simulink model "mrefrobotarm_modified_previous_y_previous_u_previous_ref"  (R2018b)
settings: Solver=FixedStepAuto  StartTime=0.0  StopTime=10  RelTol=1e-3  AbsTol=1e-6
undefined symbols (not defined in the file or in its folder): options, sfunxy2
libraries: neural x949, simulink x1
(part 8 of 31)

== system mrefrobotarm_modified_previous_y_previous_u_previous_ref/Feed-Forward Neural Network/Layer 2/Delays 1 ==
  "p{2}" : Inport  PortDimensions=60
      mask Display: e = 0.06;c1 = [120 230 180]/255;c2 = ([120 230 180]+0)/(256+128);c3 = ([120 230 180]+128)/(256+128);patch([0 1 1 0],[0 0 1 1],c1);patch([0 1 1 1-e 1-e 0+e],[0 0 1 1-e 0+e 0+e],c2);patch([0 0 1 1-e 0+e 0+e],[0 1 1 1-e 1-e 0+e],c3);plot([0 1 1 0 0],[0 0 1 1 0]);
  mux : Mux  Inputs=1
      mask Display: e = 0.06;c1 = [120 150 230]/255;c2 = ([120 150 230]+0)/383;c3 = ([120 150 230]+128)/383;patch([0 1 1 0],[0 0 1 1],c1);patch([0 1 1 1-e 1-e 0+e],[0 0 1 1-e 0+e 0+e],c2);patch([0 0 1 1-e 0+e 0+e],[0 1 1 1-e 1-e 0+e],c3);plot([0 1 1 0 0],[0 0 1 1 0]);disp('Mux')
  "pd{2,1}" : Outport
      mask Display: e = 0.06;c1 = [120 230 180]/255;c2 = ([120 230 180]+0)/(256+128);c3 = ([120 230 180]+128)/(256+128);patch([0 1 1 0],[0 0 1 1],c1);patch([0 1 1 1-e 1-e 0+e],[0 0 1 1-e 0+e 0+e],c2);patch([0 0 1 1-e 0+e 0+e],[0 1 1 1-e 1-e 0+e],c3);plot([0 1 1 0 0],[0 0 1 1 0]);
  wires:
  "p{2}"/1 -> mux/1
  mux/1 -> "pd{2,1}"/1

== system mrefrobotarm_modified_previous_y_previous_u_previous_ref/Feed-Forward Neural Network/Layer 2/LW{2,1} ==
  "ad{2,1}" : Inport  PortDimensions=60
      mask Display: e = 0.06;c1 = [120 230 180]/255;c2 = ([120 230 180]+0)/(256+128);c3 = ([120 230 180]+128)/(256+128);patch([0 1 1 0],[0 0 1 1],c1);patch([0 1 1 1-e 1-e 0+e],[0 0 1 1-e 0+e 0+e],c2);patch([0 0 1 1-e 0+e 0+e],[0 1 1 1-e 1-e 0+e],c3);plot([0 1 1 0 0],[0 0 1 1 0]);
  "IW{2,1}(1,:)'" : Constant  Value=[0.004922335615622427072712863349579492933116853237152099609375;-0.000568123825967846766103741540376859120442532002925872802734375;-0.088069540363433007623683579367934726178646087646484375;0.008040519008257716870868847536257817409932613372802734375;-1.1046255112634393302784019397222436964511871337890625;1.0155388829671150308087135272216983139514923095703125;-0.0584137446587948971910009277053177356719970703125;-0.60279808328518191817835258916602469980716705322265625;-0.002127023321206248686332518360586618655361235141754150390625;-0.702093460779070976940374748664908111095428466796875;-0.5646190112434352759152034195722080767154693603515625;0.1977466023732981081906245890422724187374114990234375;0.053988746168900279831515121031770831905305385589599609375;-0.0836139079239973381785233641494414769113063812255859375;0.000321793533986787310373356429948898949078284204006195068359375;0.01929470514180042783891622093506157398223876953125;-0.004037426007550685112812427490780464722774922847747802734375;-0.006774271389454964049925411728736435179598629474639892578125;-0.12049917647571557755004079126592841930687427520751953125;-0.274181794734965844639873466803692281246185302734375;-0.03381345636772016549631558746114023961126804351806640625;-0.084568291882440027595890796874300576746463775634765625;0.01009376083310289419492367102293428615666925907135009765625;-0.1481308970879313402502219787493231706321239471435546875;-1.83977190390720490853482260718010365962982177734375;-0.0309407696275533876384411513527084025554358959197998046875;0.2451901685169690370269535151237505488097667694091796875;0.11553958397011880598892474836247856728732585906982421875;0.004316504239658881802998990906417020596563816070556640625;0.38419726481958960118134882577578537166118621826171875;-0.036990773747104264967955344900474301539361476898193359375;0.05294928752338227961882211047850432805716991424560546875;-0.004316566647762872833971048436296769068576395511627197265625;-0.00471011047120292215828474269301295862533152103424072265625;0.86826225761141750947302853091969154775142669677734375;-0.272835736891962998829086473051575012505054473876953125;-0.0133865280367646798109770855944589129649102687835693359375;0.56412398957959453138499839042196981608867645263671875;-0.4238701061208143272551751579158008098602294921875;-0.0239428666309109867971205432013448444195091724395751953125;-1.46284474525641439157652712310664355754852294921875;-0.01846824999686343116156450605558347888290882110595703125;-1.8796503475121746351561569099430926144123077392578125;0.5565875164302613864464319703984074294567108154296875;-1.2035129714628267638687475482583977282047271728515625;-0.396624881636485737690378527986467815935611724853515625;0.374562923409318404566192839411087334156036376953125;0.228885480374885597054657182525261305272579193115234375;0.29055525212637800525072862001252360641956329345703125;-0.01447757195351602292621162604291384923271834850311279296875;-0.0176065930859190811208492277728510089218616485595703125;-0.2212805191454988718025020943969138897955417633056640625;-0.064717987937388699037910555489361286163330078125;-0.402780257895579529847651656382367946207523345947265625;0.89397582203941539091829326935112476348876953125;-0.156302033504358173221504557659500278532505035400390625;-0.0055868107216290908978439944121419102884829044342041015625;-0.34665630432465055488222560597932897508144378662109375;-0.206360303612080742130530097711016424000263214111328125;0.35959441595475760689026856198324821889400482177734375]
      mask Display: e = 0.06;c1 = [120 150 230]/255;c2 = ([120 150 230]+0)/383;c3 = ([120 150 230]+128)/383;patch([0 1 1 0],[0 0 1 1],c1);patch([0 1 1 1-e 1-e 0+e],[0 0 1 1-e 0+e 0+e],c2);patch([0 0 1 1-e 0+e 0+e],[0 1 1 1-e 1-e 0+e],c3);plot([0 1 1 0 0],[0 0 1 1 0]);disp('weights');
  Mux : Mux  Inputs=1
      mask Display: e = 0.06;c1 = [120 150 230]/255;c2 = ([120 150 230]+0)/383;c3 = ([120 150 230]+128)/383;patch([0 1 1 0],[0 0 1 1],c1);patch([0 1 1 1-e 1-e 0+e],[0 0 1 1-e 0+e 0+e],c2);patch([0 0 1 1-e 0+e 0+e],[0 1 1 1-e 1-e 0+e],c3);plot([0 1 1 0 0],[0 0 1 1 0]);disp('Mux');
  dotprod1 : neural/Weight Functions/dotprod
  "lz{2,1}" : Outport
      mask Display: e = 0.06;c1 = [120 230 180]/255;c2 = ([120 230 180]+0)/(256+128);c3 = ([120 230 180]+128)/(256+128);patch([0 1 1 0],[0 0 1 1],c1);patch([0 1 1 1-e 1-e 0+e],[0 0 1 1-e 0+e 0+e],c2);patch([0 0 1 1-e 0+e 0+e],[0 1 1 1-e 1-e 0+e],c3);plot([0 1 1 0 0],[0 0 1 1 0]);
  wires:
  "IW{2,1}(1,:)'"/1 -> dotprod1/1
  "ad{2,1}"/1 -> dotprod1/2
  dotprod1/1 -> Mux/1
  Mux/1 -> "lz{2,1}"/1

== system mrefrobotarm_modified_previous_y_previous_u_previous_ref/Feed-Forward Neural Network1/Layer 1/Delays 1 ==
  "p{1}" : Inport  PortDimensions=8
      mask Display: e = 0.06;c1 = [120 230 180]/255;c2 = ([120 230 180]+0)/(256+128);c3 = ([120 230 180]+128)/(256+128);patch([0 1 1 0],[0 0 1 1],c1);patch([0 1 1 1-e 1-e 0+e],[0 0 1 1-e 0+e 0+e],c2);patch([0 0 1 1-e 0+e 0+e],[0 1 1 1-e 1-e 0+e],c3);plot([0 1 1 0 0],[0 0 1 1 0]);
  mux : Mux  Inputs=1
      mask Display: e = 0.06;c1 = [120 150 230]/255;c2 = ([120 150 230]+0)/383;c3 = ([120 150 230]+128)/383;patch([0 1 1 0],[0 0 1 1],c1);patch([0 1 1 1-e 1-e 0+e],[0 0 1 1-e 0+e 0+e],c2);patch([0 0 1 1-e 0+e 0+e],[0 1 1 1-e 1-e 0+e],c3);plot([0 1 1 0 0],[0 0 1 1 0]);disp('Mux')
  "pd{1,1}" : Outport
      mask Display: e = 0.06;c1 = [120 230 180]/255;c2 = ([120 230 180]+0)/(256+128);c3 = ([120 230 180]+128)/(256+128);patch([0 1 1 0],[0 0 1 1],c1);patch([0 1 1 1-e 1-e 0+e],[0 0 1 1-e 0+e 0+e],c2);patch([0 0 1 1-e 0+e 0+e],[0 1 1 1-e 1-e 0+e],c3);plot([0 1 1 0 0],[0 0 1 1 0]);
  wires:
  "p{1}"/1 -> mux/1
  mux/1 -> "pd{1,1}"/1

== system mrefrobotarm_modified_previous_y_previous_u_previous_ref/Feed-Forward Neural Network1/Layer 1/IW{1,1} ==
  "pd{1,1}" : Inport  PortDimensions=8
      mask Display: e = 0.06;c1 = [120 230 180]/255;c2 = ([120 230 180]+0)/(256+128);c3 = ([120 230 180]+128)/(256+128);patch([0 1 1 0],[0 0 1 1],c1);patch([0 1 1 1-e 1-e 0+e],[0 0 1 1-e 0+e 0+e],c2);patch([0 0 1 1-e 0+e 0+e],[0 1 1 1-e 1-e 0+e],c3);plot([0 1 1 0 0],[0 0 1 1 0]);
  "IW{1,1}(1,:)'" : Constant  Value=[-0.489435165671598337855385807415586896240711212158203125;-0.59790642458332443620605545220314525067806243896484375;0.9462514542685998009119430207647383213043212890625;0.87465564536648532367735242587514221668243408203125;-1.4123419584819483230120340522262267768383026123046875;0.364318026214990597910770020462223328649997711181640625;0.476243895384673543436093723357771523296833038330078125;-0.94161424505193591638629868612042628228664398193359375]
      mask Display: e = 0.06;c1 = [120 150 230]/255;c2 = ([120 150 230]+0)/383;c3 = ([120 150 230]+128)/383;patch([0 1 1 0],[0 0 1 1],c1);patch([0 1 1 1-e 1-e 0+e],[0 0 1 1-e 0+e 0+e],c2);patch([0 0 1 1-e 0+e 0+e],[0 1 1 1-e 1-e 0+e],c3);plot([0 1 1 0 0],[0 0 1 1 0]);disp('Weights');
  "IW{1,1}(10,:)'" : Constant  Value=[0.24784818454698787082435273987357504665851593017578125;0.428137490507039142340062198854866437613964080810546875;-0.279368989082627694475746693569817580282688140869140625;0.635561926772618246417323462083004415035247802734375;-0.2661724130434099944153558681136928498744964599609375;0.84937640623256982497224498729337938129901885986328125;1.1481977763386710389426070832996629178524017333984375;0.1470300152897714152100405726741882972419261932373046875]
      mask Display: e = 0.06;c1 = [120 150 230]/255;c2 = ([120 150 230]+0)/383;c3 = ([120 150 230]+128)/383;patch([0 1 1 0],[0 0 1 1],c1);patch([0 1 1 1-e 1-e 0+e],[0 0 1 1-e 0+e 0+e],c2);patch([0 0 1 1-e 0+e 0+e],[0 1 1 1-e 1-e 0+e],c3);plot([0 1 1 0 0],[0 0 1 1 0]);disp('Weights');
  "IW{1,1}(11,:)'" : Constant  Value=[0.4509913927567001934448853717185556888580322265625;0.7052495398937128623373382652061991393566131591796875;-0.7838302343464118582261335177463479340076446533203125;1.4900741834051085543677572786691598594188690185546875;-0.527849453687423864067795875598676502704620361328125;-1.02175108583142648654984441236592829227447509765625;-0.52620304449603716445693635250790975987911224365234375;-0.6238002211724491541389170379261486232280731201171875]
      mask Display: e = 0.06;c1 = [120 150 230]/255;c2 = ([120 150 230]+0)/383;c3 = ([120 150 230]+128)/383;patch([0 1 1 0],[0 0 1 1],c1);patch([0 1 1 1-e 1-e 0+e],[0 0 1 1-e 0+e 0+e],c2);patch([0 0 1 1-e 0+e 0+e],[0 1 1 1-e 1-e 0+e],c3);plot([0 1 1 0 0],[0 0 1 1 0]);disp('Weights');
  "IW{1,1}(12,:)'" : Constant  Value=[-1.6021052877080024234857091869344003498554229736328125;-0.400230307522328410119172303893719799816608428955078125;0.77757489461041362499571505395579151809215545654296875;0.2472458939471125216602587215675157494843006134033203125;-0.1976112083793134244213973715886822901666164398193359375;0.04669389623471220662764835651614703238010406494140625;0.511283230600608984417476676753722131252288818359375;-0.469639748921519550872716308731469325721263885498046875]
      mask Display: e = 0.06;c1 = [120 150 230]/255;c2 = ([120 150 230]+0)/383;c3 = ([120 150 230]+128)/383;patch([0 1 1 0],[0 0 1 1],c1);patch([0 1 1 1-e 1-e 0+e],[0 0 1 1-e 0+e 0+e],c2);patch([0 0 1 1-e 0+e 0+e],[0 1 1 1-e 1-e 0+e],c3);plot([0 1 1 0 0],[0 0 1 1 0]);disp('Weights');
  "IW{1,1}(13,:)'" : Constant  Value=[-1.6051933424153304041936962676118128001689910888671875;-1.5266914996233234003142342771752737462520599365234375;0.332608030744975857739831326398416422307491302490234375;-0.59175031390800969521848173826583661139011383056640625;0.45672389039967864476921022287569940090179443359375;-0.1611477461390518894912560199372819624841213226318359375;0.0258266856071377344516992735634630662389099597930908203125;1.0826091475290675614218116606934927403926849365234375]
      mask Display: e = 0.06;c1 = [120 150 230]/255;c2 = ([120 150 230]+0)/383;c3 = ([120 150 230]+128)/383;patch([0 1 1 0],[0 0 1 1],c1);patch([0 1 1 1-e 1-e 0+e],[0 0 1 1-e 0+e 0+e],c2);patch([0 0 1 1-e 0+e 0+e],[0 1 1 1-e 1-e 0+e],c3);plot([0 1 1 0 0],[0 0 1 1 0]);disp('Weights');
  "IW{1,1}(14,:)'" : Constant  Value=[-0.20824009402255339029608194323373027145862579345703125;-0.63002483804711406634169179596938192844390869140625;0.6012849457953872711613030332955531775951385498046875;0.1919364347106604640202931477688252925872802734375;-0.56970968188246418062448128694086335599422454833984375;0.2051097651594903925609258976692217402160167694091796875;0.260356801348437638665700433193705976009368896484375;1.5726063671236916174933639922528527677059173583984375]
      mask Display: e = 0.06;c1 = [120 150 230]/255;c2 = ([120 150 230]+0)/383;c3 = ([120 150 230]+128)/383;patch([0 1 1 0],[0 0 1 1],c1);patch([0 1 1 1-e 1-e 0+e],[0 0 1 1-e 0+e 0+e],c2);patch([0 0 1 1-e 0+e 0+e],[0 1 1 1-e 1-e 0+e],c3);plot([0 1 1 0 0],[0 0 1 1 0]);disp('Weights');
  "IW{1,1}(15,:)'" : Constant  Value=[0.6453341252687445628311024847789667546749114990234375;-0.5310115058985160896298793886671774089336395263671875;-0.48721002209239483438096840473008342087268829345703125;-0.63616173475083803712237795480177737772464752197265625;-0.455222345196995281657592613555607385933399200439453125;-0.20214300406766472217867658400791697204113006591796875;0.85975492967386080156444450039998628199100494384765625;-0.30000078268944407877683033802895806729793548583984375]
      mask Display: e = 0.06;c1 = [120 150 230]/255;c2 = ([120 150 230]+0)/383;c3 = ([120 150 230]+128)/383;patch([0 1 1 0],[0 0 1 1],c1);patch([0 1 1 1-e 1-e 0+e],[0 0 1 1-e 0+e 0+e],c2);patch([0 0 1 1-e 0+e 0+e],[0 1 1 1-e 1-e 0+e],c3);plot([0 1 1 0 0],[0 0 1 1 0]);disp('Weights');
  "IW{1,1}(16,:)'" : Constant  Value=[-1.2705032748254423413669655928970314562320709228515625;0.460182504971557937434312179902917705476284027099609375;-0.7014528933886319261858943718834780156612396240234375;-1.3600973186092204514352488331496715545654296875;-0.380943287230387894748417920709471218287944793701171875;-0.182287628267785828395375347099616192281246185302734375;0.76493247291822685784978830270119942724704742431640625;-0.1468958452647432244564384973273263312876224517822265625]
      mask Display: e = 0.06;c1 = [120 150 230]/255;c2 = ([120 150 230]+0)/383;c3 = ([120 150 230]+128)/383;patch([0 1 1 0],[0 0 1 1],c1);patch([0 1 1 1-e 1-e 0+e],[0 0 1 1-e 0+e 0+e],c2);patch([0 0 1 1-e 0+e 0+e],[0 1 1 1-e 1-e 0+e],c3);plot([0 1 1 0 0],[0 0 1 1 0]);disp('Weights');
  "IW{1,1}(2,:)'" : Constant  Value=[0.05544360121873585789398219958457048051059246063232421875;-0.6084945450961765089914479176513850688934326171875;0.8236590711365157080336985018220730125904083251953125;0.0942136023378637166292293159131077118217945098876953125;-0.10857743809028670700644880753316101618111133575439453125;0.02981406738831320069049723997522960416972637176513671875;0.198421637732602185177910314450855366885662078857421875;1.001382968907298387506443759775720536708831787109375]
      mask Display: e = 0.06;c1 = [120 150 230]/255;c2 = ([120 150 230]+0)/383;c3 = ([120 150 230]+128)/383;patch([0 1 1 0],[0 0 1 1],c1);patch([0 1 1 1-e 1-e 0+e],[0 0 1 1-e 0+e 0+e],c2);patch([0 0 1 1-e 0+e 0+e],[0 1 1 1-e 1-e 0+e],c3);plot([0 1 1 0 0],[0 0 1 1 0]);disp('Weights');
  "IW{1,1}(3,:)'" : Constant  Value=[-0.293870924391490262461701377105782739818096160888671875;0.48987560205334046425917904343805275857448577880859375;-0.226064051583725611482833528498304076492786407470703125;0.54526247608860656246321241269470192492008209228515625;-1.0762508709854230470881475412170402705669403076171875;0.54304733376469815908649252378381788730621337890625;0.0237025381828885155222064184954433585517108440399169921875;-0.476213427298837921330942890563164837658405303955078125]
      mask Display: e = 0.06;c1 = [120 150 230]/255;c2 = ([120 150 230]+0)/383;c3 = ([120 150 230]+128)/383;patch([0 1 1 0],[0 0 1 1],c1);patch([0 1 1 1-e 1-e 0+e],[0 0 1 1-e 0+e 0+e],c2);patch([0 0 1 1-e 0+e 0+e],[0 1 1 1-e 1-e 0+e],c3);plot([0 1 1 0 0],[0 0 1 1 0]);disp('Weights');
  "IW{1,1}(4,:)'" : Constant  Value=[1.46243602440109743412222087499685585498809814453125;-0.6143515017476561812515001292922534048557281494140625;-0.813339714393659818369997083209455013275146484375;0.12431520627244212195972039580738055519759654998779296875;1.0257454781333077420413246727548539638519287109375;-1.3024201622922590981801249654381535947322845458984375;0.57650698104107267472073772296425886452198028564453125;0.20537346279362023171444207036984153091907501220703125]
      mask Display: e = 0.06;c1 = [120 150 230]/255;c2 = ([120 150 230]+0)/383;c3 = ([120 150 230]+128)/383;patch([0 1 1 0],[0 0 1 1],c1);patch([0 1 1 1-e 1-e 0+e],[0 0 1 1-e 0+e 0+e],c2);patch([0 0 1 1-e 0+e 0+e],[0 1 1 1-e 1-e 0+e],c3);plot([0 1 1 0 0],[0 0 1 1 0]);disp('Weights');
  "IW{1,1}(5,:)'" : Constant  Value=[0.2161689026789992140731300196421216242015361785888671875;-1.068678632626362201563097187317907810211181640625;0.57330147110937723642365426712785847485065460205078125;0.08697750843062114489701031061485991813242435455322265625;-0.325667357124172607285572667024098336696624755859375;-0.04243784278384317432131211944579263217747211456298828125;1.123940770278660128411729601793922483921051025390625;1.3019794387795020629283726520952768623828887939453125]
      mask Display: e = 0.06;c1 = [120 150 230]/255;c2 = ([120 150 230]+0)/383;c3 = ([120 150 230]+128)/383;patch([0 1 1 0],[0 0 1 1],c1);patch([0 1 1 1-e 1-e 0+e],[0 0 1 1-e 0+e 0+e],c2);patch([0 0 1 1-e 0+e 0+e],[0 1 1 1-e 1-e 0+e],c3);plot([0 1 1 0 0],[0 0 1 1 0]);disp('Weights');
  "IW{1,1}(6,:)'" : Constant  Value=[-1.2478069984792659052885710480040870606899261474609375;-0.1258253740427072997487556449414114467799663543701171875;-0.88679456135978573794176327282912097871303558349609375;-0.2182788795135275072833991316656465642154216766357421875;-0.7833970842850959126479892802308313548564910888671875;0.9419426170986813229291101379203610122203826904296875;-1.05803585202793914987751122680492699146270751953125;0.9246942036142489218519813221064396202564239501953125]
      mask Display: e = 0.06;c1 = [120 150 230]/255;c2 = ([120 150 230]+0)/383;c3 = ([120 150 230]+128)/383;patch([0 1 1 0],[0 0 1 1],c1);patch([0 1 1 1-e 1-e 0+e],[0 0 1 1-e 0+e 0+e],c2);patch([0 0 1 1-e 0+e 0+e],[0 1 1 1-e 1-e 0+e],c3);plot([0 1 1 0 0],[0 0 1 1 0]);disp('Weights');
  "IW{1,1}(7,:)'" : Constant  Value=[1.59052415695107551840692394762299954891204833984375;-1.407606543352498018606411278597079217433929443359375;-0.33944053433563514676762906674412079155445098876953125;-0.72464187144598124490357804461382329463958740234375;1.7120549882542188679934724859776906669139862060546875;-0.74145695282181967034063063692883588373661041259765625;0.50968036339168032444746359033160842955112457275390625;0.83650127749657865461330175094190053641796112060546875]
      mask Display: e = 0.06;c1 = [120 150 230]/255;c2 = ([120 150 230]+0)/383;c3 = ([120 150 230]+128)/383;patch([0 1 1 0],[0 0 1 1],c1);patch([0 1 1 1-e 1-e 0+e],[0 0 1 1-e 0+e 0+e],c2);patch([0 0 1 1-e 0+e 0+e],[0 1 1 1-e 1-e 0+e],c3);plot([0 1 1 0 0],[0 0 1 1 0]);disp('Weights');
  "IW{1,1}(8,:)'" : Constant  Value=[0.0659504331933596088521909450719249434769153594970703125;-0.98697499307263447665405919906334020197391510009765625;1.1401596825984083860561213441542349755764007568359375;-1.0640028818961406731347096865647472441196441650390625;-0.4904056650842238962439978422480635344982147216796875;-0.361254192958798736601266909929108805954456329345703125;-0.41512670811280916183250155881978571414947509765625;-0.43991779302995437372914011575630865991115570068359375]
      mask Display: e = 0.06;c1 = [120 150 230]/255;c2 = ([120 150 230]+0)/383;c3 = ([120 150 230]+128)/383;patch([0 1 1 0],[0 0 1 1],c1);patch([0 1 1 1-e 1-e 0+e],[0 0 1 1-e 0+e 0+e],c2);patch([0 0 1 1-e 0+e 0+e],[0 1 1 1-e 1-e 0+e],c3);plot([0 1 1 0 0],[0 0 1 1 0]);disp('Weights');
  "IW{1,1}(9,:)'" : Constant  Value=[0.9288936158440825874293977904017083346843719482421875;0.1536580527370895177252663188482983969151973724365234375;-1.1504658879815246041999898807262070477008819580078125;-0.5619971281848823441151807855931110680103302001953125;-0.304875849992781444708356275441474281251430511474609375;-0.857832390191720417504939177888445556163787841796875;0.6730201883496238490778296181815676391124725341796875;0.330856347068350709061945735811605118215084075927734375]
      mask Display: e = 0.06;c1 = [120 150 230]/255;c2 = ([120 150 230]+0)/383;c3 = ([120 150 230]+128)/383;patch([0 1 1 0],[0 0 1 1],c1);patch([0 1 1 1-e 1-e 0+e],[0 0 1 1-e 0+e 0+e],c2);patch([0 0 1 1-e 0+e 0+e],[0 1 1 1-e 1-e 0+e],c3);plot([0 1 1 0 0],[0 0 1 1 0]);disp('Weights');
  Mux : Mux  Inputs=16
      mask Display: e = 0.06;c1 = [120 150 230]/255;c2 = ([120 150 230]+0)/383;c3 = ([120 150 230]+128)/383;patch([0 1 1 0],[0 0 1 1],c1);patch([0 1 1 1-e 1-e 0+e],[0 0 1 1-e 0+e 0+e],c2);patch([0 0 1 1-e 0+e 0+e],[0 1 1 1-e 1-e 0+e],c3);plot([0 1 1 0 0],[0 0 1 1 0]);disp('Mux');
  dotprod{1..16} (16 alike) : neural/Weight Functions/dotprod
  "iz{1,1}" : Outport
      mask Display: e = 0.06;c1 = [120 230 180]/255;c2 = ([120 230 180]+0)/(256+128);c3 = ([120 230 180]+128)/(256+128);patch([0 1 1 0],[0 0 1 1],c1);patch([0 1 1 1-e 1-e 0+e],[0 0 1 1-e 0+e 0+e],c2);patch([0 0 1 1-e 0+e 0+e],[0 1 1 1-e 1-e 0+e],c3);plot([0 1 1 0 0],[0 0 1 1 0]);
  wires:
  "IW{1,1}(1,:)'"/1 -> dotprod1/1
  "pd{1,1}"/1 -> dotprod1/2, dotprod2/2, dotprod3/2, dotprod4/2, dotprod5/2, dotprod6/2, dotprod7/2, dotprod8/2, dotprod9/2, dotprod10/2, dotprod11/2, dotprod12/2, dotprod13/2, dotprod14/2, dotprod15/2, dotprod16/2
  dotprod1/1 -> Mux/1
  "IW{1,1}(2,:)'"/1 -> dotprod2/1
  dotprod2/1 -> Mux/2
  "IW{1,1}(3,:)'"/1 -> dotprod3/1
  dotprod3/1 -> Mux/3
  "IW{1,1}(4,:)'"/1 -> dotprod4/1
  dotprod4/1 -> Mux/4
  "IW{1,1}(5,:)'"/1 -> dotprod5/1
  dotprod5/1 -> Mux/5
  "IW{1,1}(6,:)'"/1 -> dotprod6/1
  dotprod6/1 -> Mux/6
  "IW{1,1}(7,:)'"/1 -> dotprod7/1
  dotprod7/1 -> Mux/7
  "IW{1,1}(8,:)'"/1 -> dotprod8/1
  dotprod8/1 -> Mux/8
  "IW{1,1}(9,:)'"/1 -> dotprod9/1
  dotprod9/1 -> Mux/9
  "IW{1,1}(10,:)'"/1 -> dotprod10/1
  dotprod10/1 -> Mux/10
  "IW{1,1}(11,:)'"/1 -> dotprod11/1
  dotprod11/1 -> Mux/11
  "IW{1,1}(12,:)'"/1 -> dotprod12/1
  dotprod12/1 -> Mux/12
  "IW{1,1}(13,:)'"/1 -> dotprod13/1
  dotprod13/1 -> Mux/13
  "IW{1,1}(14,:)'"/1 -> dotprod14/1
  dotprod14/1 -> Mux/14
  "IW{1,1}(15,:)'"/1 -> dotprod15/1
  dotprod15/1 -> Mux/15
  "IW{1,1}(16,:)'"/1 -> dotprod16/1
  dotprod16/1 -> Mux/16
  Mux/1 -> "iz{1,1}"/1

== system mrefrobotarm_modified_previous_y_previous_u_previous_ref/Feed-Forward Neural Network1/Layer 2/Delays 1 ==
  "p{2}" : Inport  PortDimensions=16
      mask Display: e = 0.06;c1 = [120 230 180]/255;c2 = ([120 230 180]+0)/(256+128);c3 = ([120 230 180]+128)/(256+128);patch([0 1 1 0],[0 0 1 1],c1);patch([0 1 1 1-e 1-e 0+e],[0 0 1 1-e 0+e 0+e],c2);patch([0 0 1 1-e 0+e 0+e],[0 1 1 1-e 1-e 0+e],c3);plot([0 1 1 0 0],[0 0 1 1 0]);
  mux : Mux  Inputs=1
      mask Display: e = 0.06;c1 = [120 150 230]/255;c2 = ([120 150 230]+0)/383;c3 = ([120 150 230]+128)/383;patch([0 1 1 0],[0 0 1 1],c1);patch([0 1 1 1-e 1-e 0+e],[0 0 1 1-e 0+e 0+e],c2);patch([0 0 1 1-e 0+e 0+e],[0 1 1 1-e 1-e 0+e],c3);plot([0 1 1 0 0],[0 0 1 1 0]);disp('Mux')
  "pd{2,1}" : Outport
      mask Display: e = 0.06;c1 = [120 230 180]/255;c2 = ([120 230 180]+0)/(256+128);c3 = ([120 230 180]+128)/(256+128);patch([0 1 1 0],[0 0 1 1],c1);patch([0 1 1 1-e 1-e 0+e],[0 0 1 1-e 0+e 0+e],c2);patch([0 0 1 1-e 0+e 0+e],[0 1 1 1-e 1-e 0+e],c3);plot([0 1 1 0 0],[0 0 1 1 0]);
  wires:
  "p{2}"/1 -> mux/1
  mux/1 -> "pd{2,1}"/1

== system mrefrobotarm_modified_previous_y_previous_u_previous_ref/Feed-Forward Neural Network1/Layer 2/LW{2,1} ==
  "ad{2,1}" : Inport  PortDimensions=16
      mask Display: e = 0.06;c1 = [120 230 180]/255;c2 = ([120 230 180]+0)/(256+128);c3 = ([120 230 180]+128)/(256+128);patch([0 1 1 0],[0 0 1 1],c1);patch([0 1 1 1-e 1-e 0+e],[0 0 1 1-e 0+e 0+e],c2);patch([0 0 1 1-e 0+e 0+e],[0 1 1 1-e 1-e 0+e],c3);plot([0 1 1 0 0],[0 0 1 1 0]);
  "IW{2,1}(1,:)'" : Constant  Value=[-0.11795628438408246874136153792278491891920566558837890625;-0.7266789733215304192270878047565929591655731201171875;-0.01225474918483036683436449010287105920724570751190185546875;1.02269129686591053740585266496054828166961669921875;0.5591836780849244181723634028458036482334136962890625;0.42706217586793082663376708296709693968296051025390625;-0.417388293832526124926829425021423958241939544677734375;-0.1721134449178444991712666478633764199912548065185546875;0.6953623528184278423935893442831002175807952880859375;0.5549726126551786098417551329475827515125274658203125;-0.75980368835832035045996235567145049571990966796875;-0.12272926696519197153900648800117778591811656951904296875;-0.42041936020313819266647215044940821826457977294921875;0.20980740921632012874198380814050324261188507080078125;-0.5296127441355171772130461249616928398609161376953125;0.2295249142940899156339895625933422707021236419677734375]
      mask Display: e = 0.06;c1 = [120 150 230]/255;c2 = ([120 150 230]+0)/383;c3 = ([120 150 230]+128)/383;patch([0 1 1 0],[0 0 1 1],c1);patch([0 1 1 1-e 1-e 0+e],[0 0 1 1-e 0+e 0+e],c2);patch([0 0 1 1-e 0+e 0+e],[0 1 1 1-e 1-e 0+e],c3);plot([0 1 1 0 0],[0 0 1 1 0]);disp('weights');
  "IW{2,1}(2,:)'" : Constant  Value=[-0.70693226414642784671826802878058515489101409912109375;0.256775847609288121464743426258792169392108917236328125;-0.94969196839098402040946211855043657124042510986328125;-0.424726446476546837249799182245624251663684844970703125;0.11347593592205339196876678897751844488084316253662109375;0.008291581221170109261553449186976649798452854156494140625;0.1784639836572024240712863729640957899391651153564453125;0.01066492483621101113044904451498950948007404804229736328125;-0.00995209252704191103811037777404635562561452388763427734375;-0.00229363338981328386545488484671295736916363239288330078125;-0.0224035193360632121917230819008182152174413204193115234375;-0.030759149339129966682637729036287055350840091705322265625;0.00075142469782060218597141698637642548419535160064697265625;0.268854822303092044766259505195193924009799957275390625;0.030060076502329953485048719130645622499287128448486328125;0.0012942506681802861019658923424913155031390488147735595703125]
      mask Display: e = 0.06;c1 = [120 150 230]/255;c2 = ([120 150 230]+0)/383;c3 = ([120 150 230]+128)/383;patch([0 1 1 0],[0 0 1 1],c1);patch([0 1 1 1-e 1-e 0+e],[0 0 1 1-e 0+e 0+e],c2);patch([0 0 1 1-e 0+e 0+e],[0 1 1 1-e 1-e 0+e],c3);plot([0 1 1 0 0],[0 0 1 1 0]);disp('weights');
  "IW{2,1}(3,:)'" : Constant  Value=[-0.177218403680896530172361735822050832211971282958984375;-1.6435982186071356192513803762267343699932098388671875;-0.365543489992732950621956433678860776126384735107421875;-0.64029549655489381709827512167976237833499908447265625;-0.05527517403068492318762849890845245681703090667724609375;-0.0192559918460919743399273329487186856567859649658203125;-0.79638903063763155643073332612402737140655517578125;-0.568818099993506631761874814401380717754364013671875;0.3713061862740374419189492982695810496807098388671875;0.1303239076645476279825430765413329936563968658447265625;0.091426230001879604802894618842401541769504547119140625;0.280553739252684675165028238552622497081756591796875;-0.1643575122097340746041282955047790892422199249267578125;-0.74487261476522814707124098276835866272449493408203125;0.44181976907313791347320375280105508863925933837890625;0.6268588315218976969589448344777338206768035888671875]
      mask Display: e = 0.06;c1 = [120 150 230]/255;c2 = ([120 150 230]+0)/383;c3 = ([120 150 230]+128)/383;patch([0 1 1 0],[0 0 1 1],c1);patch([0 1 1 1-e 1-e 0+e],[0 0 1 1-e 0+e 0+e],c2);patch([0 0 1 1-e 0+e 0+e],[0 1 1 1-e 1-e 0+e],c3);plot([0 1 1 0 0],[0 0 1 1 0]);disp('weights');
  "IW{2,1}(4,:)'" : Constant  Value=[-0.7454559855908058363382906463812105357646942138671875;-0.1806292113311284974752624066240969114005565643310546875;-0.54735698289510048564210364929749630391597747802734375;0.7599786448544338934851793965208344161510467529296875;0.83126805597514608070497388325748033821582794189453125;0.11427376477351146311089991058906889520585536956787109375;1.2631282692396996747419279927271418273448944091796875;0.309484415009570079657663654870702885091304779052734375;0.490505612211509511855211940201115794479846954345703125;-0.350154579470569993215889326165779493749141693115234375;-1.2363135611592117601986728914198465645313262939453125;0.0009064516084202668168290362160632867016829550266265869140625;-1.0378501856620532262098777209757827222347259521484375;0.474155328660954278330308397926273755729198455810546875;-0.503012773734166085404240220668725669384002685546875;0.33278231968638360971368683749460615217685699462890625]
      mask Display: e = 0.06;c1 = [120 150 230]/255;c2 = ([120 150 230]+0)/383;c3 = ([120 150 230]+128)/383;patch([0 1 1 0],[0 0 1 1],c1);patch([0 1 1 1-e 1-e 0+e],[0 0 1 1-e 0+e 0+e],c2);patch([0 0 1 1-e 0+e 0+e],[0 1 1 1-e 1-e 0+e],c3);plot([0 1 1 0 0],[0 0 1 1 0]);disp('weights');
  Mux : Mux
      mask Display: e = 0.06;c1 = [120 150 230]/255;c2 = ([120 150 230]+0)/383;c3 = ([120 150 230]+128)/383;patch([0 1 1 0],[0 0 1 1],c1);patch([0 1 1 1-e 1-e 0+e],[0 0 1 1-e 0+e 0+e],c2);patch([0 0 1 1-e 0+e 0+e],[0 1 1 1-e 1-e 0+e],c3);plot([0 1 1 0 0],[0 0 1 1 0]);disp('Mux');
  dotprod{1..4} (4 alike) : neural/Weight Functions/dotprod
  "lz{2,1}" : Outport
      mask Display: e = 0.06;c1 = [120 230 180]/255;c2 = ([120 230 180]+0)/(256+128);c3 = ([120 230 180]+128)/(256+128);patch([0 1 1 0],[0 0 1 1],c1);patch([0 1 1 1-e 1-e 0+e],[0 0 1 1-e 0+e 0+e],c2);patch([0 0 1 1-e 0+e 0+e],[0 1 1 1-e 1-e 0+e],c3);plot([0 1 1 0 0],[0 0 1 1 0]);
  wires:
  "IW{2,1}(1,:)'"/1 -> dotprod1/1
  "ad{2,1}"/1 -> dotprod1/2, dotprod2/2, dotprod3/2, dotprod4/2
  dotprod1/1 -> Mux/1
  "IW{2,1}(2,:)'"/1 -> dotprod2/1
  dotprod2/1 -> Mux/2
  "IW{2,1}(3,:)'"/1 -> dotprod3/1
  dotprod3/1 -> Mux/3
  "IW{2,1}(4,:)'"/1 -> dotprod4/1
  dotprod4/1 -> Mux/4
  Mux/1 -> "lz{2,1}"/1

== system mrefrobotarm_modified_previous_y_previous_u_previous_ref/Feed-Forward Neural Network1/Layer 3/Delays 1 ==
  "p{3}" : Inport  PortDimensions=4
      mask Display: e = 0.06;c1 = [120 230 180]/255;c2 = ([120 230 180]+0)/(256+128);c3 = ([120 230 180]+128)/(256+128);patch([0 1 1 0],[0 0 1 1],c1);patch([0 1 1 1-e 1-e 0+e],[0 0 1 1-e 0+e 0+e],c2);patch([0 0 1 1-e 0+e 0+e],[0 1 1 1-e 1-e 0+e],c3);plot([0 1 1 0 0],[0 0 1 1 0]);
  mux : Mux  Inputs=1
      mask Display: e = 0.06;c1 = [120 150 230]/255;c2 = ([120 150 230]+0)/383;c3 = ([120 150 230]+128)/383;patch([0 1 1 0],[0 0 1 1],c1);patch([0 1 1 1-e 1-e 0+e],[0 0 1 1-e 0+e 0+e],c2);patch([0 0 1 1-e 0+e 0+e],[0 1 1 1-e 1-e 0+e],c3);plot([0 1 1 0 0],[0 0 1 1 0]);disp('Mux')
  "pd{3,2}" : Outport
      mask Display: e = 0.06;c1 = [120 230 180]/255;c2 = ([120 230 180]+0)/(256+128);c3 = ([120 230 180]+128)/(256+128);patch([0 1 1 0],[0 0 1 1],c1);patch([0 1 1 1-e 1-e 0+e],[0 0 1 1-e 0+e 0+e],c2);patch([0 0 1 1-e 0+e 0+e],[0 1 1 1-e 1-e 0+e],c3);plot([0 1 1 0 0],[0 0 1 1 0]);
  wires:
  "p{3}"/1 -> mux/1
  mux/1 -> "pd{3,2}"/1

== system mrefrobotarm_modified_previous_y_previous_u_previous_ref/Feed-Forward Neural Network1/Layer 3/LW{3,2} ==
  "ad{3,2}" : Inport  PortDimensions=4
      mask Display: e = 0.06;c1 = [120 230 180]/255;c2 = ([120 230 180]+0)/(256+128);c3 = ([120 230 180]+128)/(256+128);patch([0 1 1 0],[0 0 1 1],c1);patch([0 1 1 1-e 1-e 0+e],[0 0 1 1-e 0+e 0+e],c2);patch([0 0 1 1-e 0+e 0+e],[0 1 1 1-e 1-e 0+e],c3);plot([0 1 1 0 0],[0 0 1 1 0]);
  "IW{3,2}(1,:)'" : Constant  Value=[-0.8539034967679299814591331596602685749530792236328125;1.09024610933651100452834725729189813137054443359375;-0.03959408350371797224998005049201310612261295318603515625;0.76830465253955981808076103334315121173858642578125]
      mask Display: e = 0.06;c1 = [120 150 230]/255;c2 = ([120 150 230]+0)/383;c3 = ([120 150 230]+128)/383;patch([0 1 1 0],[0 0 1 1],c1);patch([0 1 1 1-e 1-e 0+e],[0 0 1 1-e 0+e 0+e],c2);patch([0 0 1 1-e 0+e 0+e],[0 1 1 1-e 1-e 0+e],c3);plot([0 1 1 0 0],[0 0 1 1 0]);disp('weights');
  Mux : Mux  Inputs=1
      mask Display: e = 0.06;c1 = [120 150 230]/255;c2 = ([120 150 230]+0)/383;c3 = ([120 150 230]+128)/383;patch([0 1 1 0],[0 0 1 1],c1);patch([0 1 1 1-e 1-e 0+e],[0 0 1 1-e 0+e 0+e],c2);patch([0 0 1 1-e 0+e 0+e],[0 1 1 1-e 1-e 0+e],c3);plot([0 1 1 0 0],[0 0 1 1 0]);disp('Mux');
  dotprod1 : neural/Weight Functions/dotprod
  "lz{3,2}" : Outport
      mask Display: e = 0.06;c1 = [120 230 180]/255;c2 = ([120 230 180]+0)/(256+128);c3 = ([120 230 180]+128)/(256+128);patch([0 1 1 0],[0 0 1 1],c1);patch([0 1 1 1-e 1-e 0+e],[0 0 1 1-e 0+e 0+e],c2);patch([0 0 1 1-e 0+e 0+e],[0 1 1 1-e 1-e 0+e],c3);plot([0 1 1 0 0],[0 0 1 1 0]);
  wires:
  "IW{3,2}(1,:)'"/1 -> dotprod1/1
  "ad{3,2}"/1 -> dotprod1/2
  dotprod1/1 -> Mux/1
  Mux/1 -> "lz{3,2}"/1

== system mrefrobotarm_modified_previous_y_previous_u_previous_ref/Feed-Forward Neural Network2/Layer 1/Delays 1 ==
  "p{1}" : Inport  PortDimensions=8
      mask Display: e = 0.06;c1 = [120 230 180]/255;c2 = ([120 230 180]+0)/(256+128);c3 = ([120 230 180]+128)/(256+128);patch([0 1 1 0],[0 0 1 1],c1);patch([0 1 1 1-e 1-e 0+e],[0 0 1 1-e 0+e 0+e],c2);patch([0 0 1 1-e 0+e 0+e],[0 1 1 1-e 1-e 0+e],c3);plot([0 1 1 0 0],[0 0 1 1 0]);
  mux : Mux  Inputs=1
      mask Display: e = 0.06;c1 = [120 150 230]/255;c2 = ([120 150 230]+0)/383;c3 = ([120 150 230]+128)/383;patch([0 1 1 0],[0 0 1 1],c1);patch([0 1 1 1-e 1-e 0+e],[0 0 1 1-e 0+e 0+e],c2);patch([0 0 1 1-e 0+e 0+e],[0 1 1 1-e 1-e 0+e],c3);plot([0 1 1 0 0],[0 0 1 1 0]);disp('Mux')
  "pd{1,1}" : Outport
      mask Display: e = 0.06;c1 = [120 230 180]/255;c2 = ([120 230 180]+0)/(256+128);c3 = ([120 230 180]+128)/(256+128);patch([0 1 1 0],[0 0 1 1],c1);patch([0 1 1 1-e 1-e 0+e],[0 0 1 1-e 0+e 0+e],c2);patch([0 0 1 1-e 0+e 0+e],[0 1 1 1-e 1-e 0+e],c3);plot([0 1 1 0 0],[0 0 1 1 0]);
  wires:
  "p{1}"/1 -> mux/1
  mux/1 -> "pd{1,1}"/1

== system mrefrobotarm_modified_previous_y_previous_u_previous_ref/Feed-Forward Neural Network2/Layer 1/IW{1,1} ==
  "pd{1,1}" : Inport  PortDimensions=8
      mask Display: e = 0.06;c1 = [120 230 180]/255;c2 = ([120 230 180]+0)/(256+128);c3 = ([120 230 180]+128)/(256+128);patch([0 1 1 0],[0 0 1 1],c1);patch([0 1 1 1-e 1-e 0+e],[0 0 1 1-e 0+e 0+e],c2);patch([0 0 1 1-e 0+e 0+e],[0 1 1 1-e 1-e 0+e],c3);plot([0 1 1 0 0],[0 0 1 1 0]);
  "IW{1,1}(1,:)'" : Constant  Value=[-1.0896782249808210085717519177705980837345123291015625;-0.503732082865798957982406136579811573028564453125;0.46177185684601107507063488810672424733638763427734375;1.2907283367527793149776016434771008789539337158203125;0.8628404996305312213422666900441981852054595947265625;-0.5778247336084152419033443948137573897838592529296875;0.95484917018315373926640177160152234137058258056640625;0.1499012305377249443250065041866037063300609588623046875]
      mask Display: e = 0.06;c1 = [120 150 230]/255;c2 = ([120 150 230]+0)/383;c3 = ([120 150 230]+128)/383;patch([0 1 1 0],[0 0 1 1],c1);patch([0 1 1 1-e 1-e 0+e],[0 0 1 1-e 0+e 0+e],c2);patch([0 0 1 1-e 0+e 0+e],[0 1 1 1-e 1-e 0+e],c3);plot([0 1 1 0 0],[0 0 1 1 0]);disp('Weights');
  "IW{1,1}(10,:)'" : Constant  Value=[0.91377866464282941905139523441903293132781982421875;0.70797825359879340556545912477304227650165557861328125;0.382797024240748129386702203191816806793212890625;0.316087995801745569313112582676694728434085845947265625;0.164557931672933477340592389737139455974102020263671875;-1.191069692984400685276114018051885068416595458984375;0.280041454964746028277744471779442392289638519287109375;1.68112811540107021102130602230317890644073486328125]
      mask Display: e = 0.06;c1 = [120 150 230]/255;c2 = ([120 150 230]+0)/383;c3 = ([120 150 230]+128)/383;patch([0 1 1 0],[0 0 1 1],c1);patch([0 1 1 1-e 1-e 0+e],[0 0 1 1-e 0+e 0+e],c2);patch([0 0 1 1-e 0+e 0+e],[0 1 1 1-e 1-e 0+e],c3);plot([0 1 1 0 0],[0 0 1 1 0]);disp('Weights');
  "IW{1,1}(11,:)'" : Constant  Value=[-0.0501759257609501185815048529548221267759799957275390625;-0.327967679411266754829767933188122697174549102783203125;0.42851406919279444451831295737065374851226806640625;0.212754145103897673863002637517638504505157470703125;-0.5456997102037977054322936965036205947399139404296875;0.2124135341597568615856772566985455341637134552001953125;0.31113924406051263193972999943071044981479644775390625;0.92191318088896689886269086855463683605194091796875]
      mask Display: e = 0.06;c1 = [120 150 230]/255;c2 = ([120 150 230]+0)/383;c3 = ([120 150 230]+128)/383;patch([0 1 1 0],[0 0 1 1],c1);patch([0 1 1 1-e 1-e 0+e],[0 0 1 1-e 0+e 0+e],c2);patch([0 0 1 1-e 0+e 0+e],[0 1 1 1-e 1-e 0+e],c3);plot([0 1 1 0 0],[0 0 1 1 0]);disp('Weights');
  "IW{1,1}(12,:)'" : Constant  Value=[-0.3850282010856405090493126408546231687068939208984375;-0.03592068021917012299315530299281817860901355743408203125;-0.2041009523528064806274784359629848040640354156494140625;-0.664305242693947750609595459536649286746978759765625;-1.086072114292379264810506356297992169857025146484375;-0.50437244999738339856776292435824871063232421875;1.218640053146353263713308479054830968379974365234375;0.07169896691572615055054740196283091790974140167236328125]
      mask Display: e = 0.06;c1 = [120 150 230]/255;c2 = ([120 150 230]+0)/383;c3 = ([120 150 230]+128)/383;patch([0 1 1 0],[0 0 1 1],c1);patch([0 1 1 1-e 1-e 0+e],[0 0 1 1-e 0+e 0+e],c2);patch([0 0 1 1-e 0+e 0+e],[0 1 1 1-e 1-e 0+e],c3);plot([0 1 1 0 0],[0 0 1 1 0]);disp('Weights');
  "IW{1,1}(13,:)'" : Constant  Value=[1.1869734433823693198206683518947102129459381103515625;-1.4890505731403933520340387985925190150737762451171875;-0.34960474758288995200672388818929903209209442138671875;0.77737519931089693603354362494428642094135284423828125;0.440774930287862132249898650115937925875186920166015625;0.1593388654841198237566146644894615747034549713134765625;-0.2425254393927148421905570785384043119847774505615234375;-0.81516450728105172007786904941895045340061187744140625]
      mask Display: e = 0.06;c1 = [120 150 230]/255;c2 = ([120 150 230]+0)/383;c3 = ([120 150 230]+128)/383;patch([0 1 1 0],[0 0 1 1],c1);patch([0 1 1 1-e 1-e 0+e],[0 0 1 1-e 0+e 0+e],c2);patch([0 0 1 1-e 0+e 0+e],[0 1 1 1-e 1-e 0+e],c3);plot([0 1 1 0 0],[0 0 1 1 0]);disp('Weights');
  "IW{1,1}(14,:)'" : Constant  Value=[-1.2894153754636110686959682425367645919322967529296875;-0.94284247732387871376857901850598864257335662841796875;0.90115381249514026062996663313242606818675994873046875;-0.371007867094769017146660416983650065958499908447265625;-0.6148865342275879886102529781055636703968048095703125;0.9512203983454359246252352022565901279449462890625;0.64472477621669910252677482276340015232563018798828125;-0.41065146133101759762240590134751982986927032470703125]
      mask Display: e = 0.06;c1 = [120 150 230]/255;c2 = ([120 150 230]+0)/383;c3 = ([120 150 230]+128)/383;patch([0 1 1 0],[0 0 1 1],c1);patch([0 1 1 1-e 1-e 0+e],[0 0 1 1-e 0+e 0+e],c2);patch([0 0 1 1-e 0+e 0+e],[0 1 1 1-e 1-e 0+e],c3);plot([0 1 1 0 0],[0 0 1 1 0]);disp('Weights');
  "IW{1,1}(15,:)'" : Constant  Value=[0.55785202451898141529085251022479496896266937255859375;-0.0448678277161593530575345312172430567443370819091796875;0.42355564503483933425087570867617614567279815673828125;-0.44219942586643645743293973282561637461185455322265625;0.120728713829701572723962499367189593613147735595703125;-1.428381323262932323103768794680945575237274169921875;-0.1335947933985340563278754189013852737843990325927734375;0.5666223834697581285269052386865951120853424072265625]
      mask Display: e = 0.06;c1 = [120 150 230]/255;c2 = ([120 150 230]+0)/383;c3 = ([120 150 230]+128)/383;patch([0 1 1 0],[0 0 1 1],c1);patch([0 1 1 1-e 1-e 0+e],[0 0 1 1-e 0+e 0+e],c2);patch([0 0 1 1-e 0+e 0+e],[0 1 1 1-e 1-e 0+e],c3);plot([0 1 1 0 0],[0 0 1 1 0]);disp('Weights');
  "IW{1,1}(16,:)'" : Constant  Value=[-0.265994996646676085116922649831394664943218231201171875;0.88038116794127063702291025037993676960468292236328125;0.457903975140497021545371580941719003021717071533203125;1.03686456565328111167900715372525155544281005859375;-0.413744205617428140175917405940708704292774200439453125;0.413445838387245745426668008803972043097019195556640625;-1.1993071302647140274899584255763329565525054931640625;0.5544209196555567320530144570511765778064727783203125]
      mask Display: e = 0.06;c1 = [120 150 230]/255;c2 = ([120 150 230]+0)/383;c3 = ([120 150 230]+128)/383;patch([0 1 1 0],[0 0 1 1],c1);patch([0 1 1 1-e 1-e 0+e],[0 0 1 1-e 0+e 0+e],c2);patch([0 0 1 1-e 0+e 0+e],[0 1 1 1-e 1-e 0+e],c3);plot([0 1 1 0 0],[0 0 1 1 0]);disp('Weights');
  "IW{1,1}(2,:)'" : Constant  Value=[0.18509426728151490149087976533337496221065521240234375;0.3293631527428437788529436147655360400676727294921875;0.416993283048705587479076939416700042784214019775390625;-0.336590309467502624141133082957821898162364959716796875;-0.824869660611103672209765136358328163623809814453125;1.0833657851167528551883378895581699907779693603515625;-1.19078186813195685544997104443609714508056640625;-0.134030160560445532613726982162916101515293121337890625]
      mask Display: e = 0.06;c1 = [120 150 230]/255;c2 = ([120 150 230]+0)/383;c3 = ([120 150 230]+128)/383;patch([0 1 1 0],[0 0 1 1],c1);patch([0 1 1 1-e 1-e 0+e],[0 0 1 1-e 0+e 0+e],c2);patch([0 0 1 1-e 0+e 0+e],[0 1 1 1-e 1-e 0+e],c3);plot([0 1 1 0 0],[0 0 1 1 0]);disp('Weights');
  "IW{1,1}(3,:)'" : Constant  Value=[-0.046451124239469239463051764005285804159939289093017578125;1.174294816601300084357717423699796199798583984375;0.2330876722373442788693864713422954082489013671875;-0.01104191827853419176352911534877421217970550060272216796875;-0.364817787935423243350641087090480141341686248779296875;-0.933113944959905960985224737669341266155242919921875;-0.74154367112909824744093612025608308613300323486328125;0.80514882799001841195973838694044388830661773681640625]
      mask Display: e = 0.06;c1 = [120 150 230]/255;c2 = ([120 150 230]+0)/383;c3 = ([120 150 230]+128)/383;patch([0 1 1 0],[0 0 1 1],c1);patch([0 1 1 1-e 1-e 0+e],[0 0 1 1-e 0+e 0+e],c2);patch([0 0 1 1-e 0+e 0+e],[0 1 1 1-e 1-e 0+e],c3);plot([0 1 1 0 0],[0 0 1 1 0]);disp('Weights');
  "IW{1,1}(4,:)'" : Constant  Value=[-0.7180316547412715078024803005973808467388153076171875;-0.4548934228217100805835571009083651006221771240234375;0.287403130340123158514842316435533575713634490966796875;1.2556680687887411540515358865377493202686309814453125;-0.08341697602347157569635527352147619239985942840576171875;0.4942646910188355224846645796787925064563751220703125;-1.1153597039299818494129112877999432384967803955078125;-0.2341785580689305923396403841252322308719158172607421875]
      mask Display: e = 0.06;c1 = [120 150 230]/255;c2 = ([120 150 230]+0)/383;c3 = ([120 150 230]+128)/383;patch([0 1 1 0],[0 0 1 1],c1);patch([0 1 1 1-e 1-e 0+e],[0 0 1 1-e 0+e 0+e],c2);patch([0 0 1 1-e 0+e 0+e],[0 1 1 1-e 1-e 0+e],c3);plot([0 1 1 0 0],[0 0 1 1 0]);disp('Weights');
  "IW{1,1}(5,:)'" : Constant  Value=[-0.0131698712420588413818389739162739715538918972015380859375;0.42305812523963937099580334688653238117694854736328125;-0.82188868403591264222285417417879216372966766357421875;0.62737416943382962042363715227111242711544036865234375;-0.92143042561298649228973545177723281085491180419921875;0.524898845222787624464899636222980916500091552734375;0.810507949620977274918232069467194378376007080078125;-1.090031339370958196610672530368901789188385009765625]
      mask Display: e = 0.06;c1 = [120 150 230]/255;c2 = ([120 150 230]+0)/383;c3 = ([120 150 230]+128)/383;patch([0 1 1 0],[0 0 1 1],c1);patch([0 1 1 1-e 1-e 0+e],[0 0 1 1-e 0+e 0+e],c2);patch([0 0 1 1-e 0+e 0+e],[0 1 1 1-e 1-e 0+e],c3);plot([0 1 1 0 0],[0 0 1 1 0]);disp('Weights');
  "IW{1,1}(6,:)'" : Constant  Value=[1.1792752604014278272615001696976833045482635498046875;-1.1206159868222560493933315228787250816822052001953125;0.3828866780886339693523723326507024466991424560546875;0.53138043772799647967985947616398334503173828125;-0.28880861289860948470931134579586796462535858154296875;0.79516330822080039109067683966713957488536834716796875;0.0990778272476224575182612852586316876113414764404296875;0.44124976342730770628719483283930458128452301025390625]
      mask Display: e = 0.06;c1 = [120 150 230]/255;c2 = ([120 150 230]+0)/383;c3 = ([120 150 230]+128)/383;patch([0 1 1 0],[0 0 1 1],c1);patch([0 1 1 1-e 1-e 0+e],[0 0 1 1-e 0+e 0+e],c2);patch([0 0 1 1-e 0+e 0+e],[0 1 1 1-e 1-e 0+e],c3);plot([0 1 1 0 0],[0 0 1 1 0]);disp('Weights');
  "IW{1,1}(7,:)'" : Constant  Value=[0.38366422668884514468601309999939985573291778564453125;0.2451224383294741404615280089274165220558643341064453125;0.358021020234488174249776193391880951821804046630859375;-1.00761348363729741350880431127734482288360595703125;1.257770545498239744830470954184420406818389892578125;-0.2694550030446645205728373184683732688426971435546875;-0.51436210162283757529877448178012855350971221923828125;0.371490509622617093299368207226507365703582763671875]
      mask Display: e = 0.06;c1 = [120 150 230]/255;c2 = ([120 150 230]+0)/383;c3 = ([120 150 230]+128)/383;patch([0 1 1 0],[0 0 1 1],c1);patch([0 1 1 1-e 1-e 0+e],[0 0 1 1-e 0+e 0+e],c2);patch([0 0 1 1-e 0+e 0+e],[0 1 1 1-e 1-e 0+e],c3);plot([0 1 1 0 0],[0 0 1 1 0]);disp('Weights');
  "IW{1,1}(8,:)'" : Constant  Value=[0.2270856745079706529022445238297223113477230072021484375;0.8952002694438083718608822891837917268276214599609375;0.3029593492990978464973750305944122374057769775390625;-0.413868045985654742224824076402001082897186279296875;-0.81938235496646039113244341933750547468662261962890625;0.61308319924496046393613823966006748378276824951171875;0.49394196254239963739252061714068986475467681884765625;-0.9824018498803521737272603786550462245941162109375]
      mask Display: e = 0.06;c1 = [120 150 230]/255;c2 = ([120 150 230]+0)/383;c3 = ([120 150 230]+128)/383;patch([0 1 1 0],[0 0 1 1],c1);patch([0 1 1 1-e 1-e 0+e],[0 0 1 1-e 0+e 0+e],c2);patch([0 0 1 1-e 0+e 0+e],[0 1 1 1-e 1-e 0+e],c3);plot([0 1 1 0 0],[0 0 1 1 0]);disp('Weights');
  "IW{1,1}(9,:)'" : Constant  Value=[-1.6275797736738824017521665155072696506977081298828125;1.47944400650204688218991577741689980030059814453125;-0.278718594866931734799209152697585523128509521484375;0.1945991159806247650099209067775518633425235748291015625;-1.2258305208119761875451558807981200516223907470703125;-0.0268262970692592465915549126975747640244662761688232421875;-0.2424049298216806314076876560648088343441486358642578125;-0.6660389583959955839276290134876035153865814208984375]
      mask Display: e = 0.06;c1 = [120 150 230]/255;c2 = ([120 150 230]+0)/383;c3 = ([120 150 230]+128)/383;patch([0 1 1 0],[0 0 1 1],c1);patch([0 1 1 1-e 1-e 0+e],[0 0 1 1-e 0+e 0+e],c2);patch([0 0 1 1-e 0+e 0+e],[0 1 1 1-e 1-e 0+e],c3);plot([0 1 1 0 0],[0 0 1 1 0]);disp('Weights');
  Mux : Mux  Inputs=16
      mask Display: e = 0.06;c1 = [120 150 230]/255;c2 = ([120 150 230]+0)/383;c3 = ([120 150 230]+128)/383;patch([0 1 1 0],[0 0 1 1],c1);patch([0 1 1 1-e 1-e 0+e],[0 0 1 1-e 0+e 0+e],c2);patch([0 0 1 1-e 0+e 0+e],[0 1 1 1-e 1-e 0+e],c3);plot([0 1 1 0 0],[0 0 1 1 0]);disp('Mux');
  dotprod{1..16} (16 alike) : neural/Weight Functions/dotprod
  "iz{1,1}" : Outport
      mask Display: e = 0.06;c1 = [120 230 180]/255;c2 = ([120 230 180]+0)/(256+128);c3 = ([120 230 180]+128)/(256+128);patch([0 1 1 0],[0 0 1 1],c1);patch([0 1 1 1-e 1-e 0+e],[0 0 1 1-e 0+e 0+e],c2);patch([0 0 1 1-e 0+e 0+e],[0 1 1 1-e 1-e 0+e],c3);plot([0 1 1 0 0],[0 0 1 1 0]);
  wires:
  "IW{1,1}(1,:)'"/1 -> dotprod1/1
  "pd{1,1}"/1 -> dotprod1/2, dotprod2/2, dotprod3/2, dotprod4/2, dotprod5/2, dotprod6/2, dotprod7/2, dotprod8/2, dotprod9/2, dotprod10/2, dotprod11/2, dotprod12/2, dotprod13/2, dotprod14/2, dotprod15/2, dotprod16/2
  dotprod1/1 -> Mux/1
  "IW{1,1}(2,:)'"/1 -> dotprod2/1
  dotprod2/1 -> Mux/2
  "IW{1,1}(3,:)'"/1 -> dotprod3/1
  dotprod3/1 -> Mux/3
  "IW{1,1}(4,:)'"/1 -> dotprod4/1
  dotprod4/1 -> Mux/4
  "IW{1,1}(5,:)'"/1 -> dotprod5/1
  dotprod5/1 -> Mux/5
  "IW{1,1}(6,:)'"/1 -> dotprod6/1
  dotprod6/1 -> Mux/6
  "IW{1,1}(7,:)'"/1 -> dotprod7/1
  dotprod7/1 -> Mux/7
  "IW{1,1}(8,:)'"/1 -> dotprod8/1
  dotprod8/1 -> Mux/8
  "IW{1,1}(9,:)'"/1 -> dotprod9/1
  dotprod9/1 -> Mux/9
  "IW{1,1}(10,:)'"/1 -> dotprod10/1
  dotprod10/1 -> Mux/10
  "IW{1,1}(11,:)'"/1 -> dotprod11/1
  dotprod11/1 -> Mux/11
  "IW{1,1}(12,:)'"/1 -> dotprod12/1
  dotprod12/1 -> Mux/12
  "IW{1,1}(13,:)'"/1 -> dotprod13/1
  dotprod13/1 -> Mux/13
  "IW{1,1}(14,:)'"/1 -> dotprod14/1
  dotprod14/1 -> Mux/14
  "IW{1,1}(15,:)'"/1 -> dotprod15/1
  dotprod15/1 -> Mux/15
  "IW{1,1}(16,:)'"/1 -> dotprod16/1
  dotprod16/1 -> Mux/16
  Mux/1 -> "iz{1,1}"/1

== system mrefrobotarm_modified_previous_y_previous_u_previous_ref/Feed-Forward Neural Network2/Layer 2/Delays 1 ==
  "p{2}" : Inport  PortDimensions=16
      mask Display: e = 0.06;c1 = [120 230 180]/255;c2 = ([120 230 180]+0)/(256+128);c3 = ([120 230 180]+128)/(256+128);patch([0 1 1 0],[0 0 1 1],c1);patch([0 1 1 1-e 1-e 0+e],[0 0 1 1-e 0+e 0+e],c2);patch([0 0 1 1-e 0+e 0+e],[0 1 1 1-e 1-e 0+e],c3);plot([0 1 1 0 0],[0 0 1 1 0]);
  mux : Mux  Inputs=1
      mask Display: e = 0.06;c1 = [120 150 230]/255;c2 = ([120 150 230]+0)/383;c3 = ([120 150 230]+128)/383;patch([0 1 1 0],[0 0 1 1],c1);patch([0 1 1 1-e 1-e 0+e],[0 0 1 1-e 0+e 0+e],c2);patch([0 0 1 1-e 0+e 0+e],[0 1 1 1-e 1-e 0+e],c3);plot([0 1 1 0 0],[0 0 1 1 0]);disp('Mux')
  "pd{2,1}" : Outport
      mask Display: e = 0.06;c1 = [120 230 180]/255;c2 = ([120 230 180]+0)/(256+128);c3 = ([120 230 180]+128)/(256+128);patch([0 1 1 0],[0 0 1 1],c1);patch([0 1 1 1-e 1-e 0+e],[0 0 1 1-e 0+e 0+e],c2);patch([0 0 1 1-e 0+e 0+e],[0 1 1 1-e 1-e 0+e],c3);plot([0 1 1 0 0],[0 0 1 1 0]);
  wires:
  "p{2}"/1 -> mux/1
  mux/1 -> "pd{2,1}"/1
